simulink model "ModeloMotorMaxon"  (R2022b)
settings: Solver=VariableStepAuto  StartTime=0.0  StopTime=60  RelTol=1e-3
libraries: cstblocks x1, slident x1
settings Model: Creator=workstation  LastModifiedBy=workstation

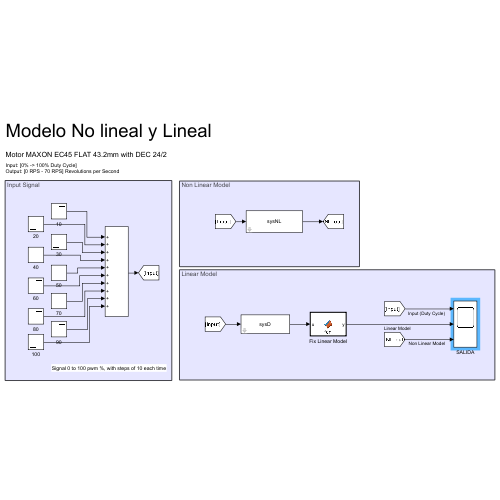
[thumbnail: Simulink's stored preview of the top-level diagram]
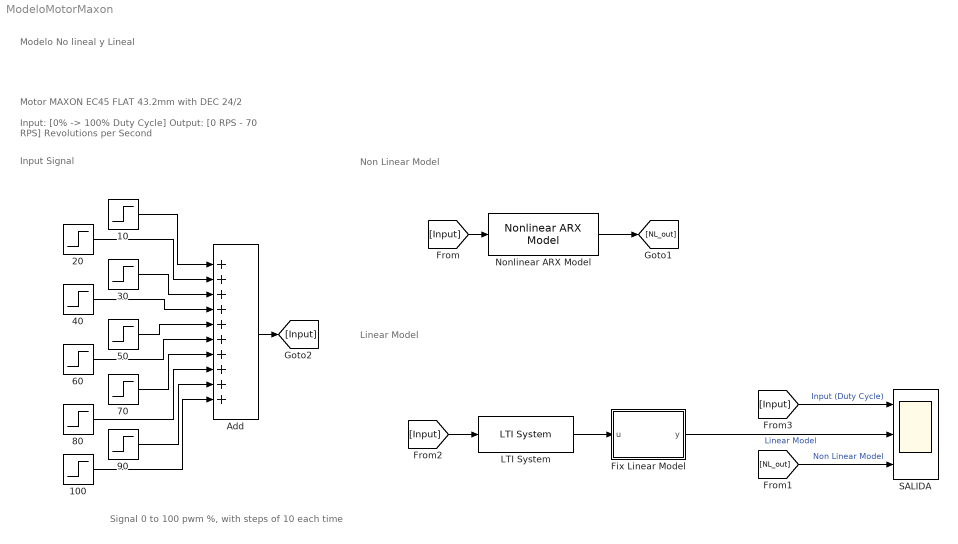
== system ModeloMotorMaxon ==
  note: Input: [0% -> 100% Duty Cycle]
      | Output: [0 RPS - 70 RPS] Revolutions per Second
  note: Signal 0 to 100 pwm %, with steps of 10 each time
  note: Input Signal
  note: Linear Model
  note: Non Linear Model
  note: Motor MAXON EC45 FLAT 43.2mm with DEC 24/2
  note: Modelo No lineal y Lineal
  10 : Step  Time=5  After=10  SampleTime=0
  100 : Step  Time=50  After=10  SampleTime=0
  20 : Step  Time=10  After=10  SampleTime=0
  30 : Step  Time=15  After=10  SampleTime=0
  40 : Step  Time=20  After=10  SampleTime=0
  50 : Step  Time=25  After=10  SampleTime=0
  60 : Step  Time=30  After=10  SampleTime=0
  70 : Step  Time=35  After=10  SampleTime=0
  80 : Step  Time=40  After=10  SampleTime=0
  90 : Step  Time=45  After=10  SampleTime=0
  Add : Sum  Inputs=++++++++++
  Fix Linear Model : MATLAB Function  TreatAsAtomicUnit=on
  LTI System : cstblocks/LTI System  sys=sysD  IC=[]
  Nonlinear ARX Model : slident/Models/Nonlinear ARX Model  sys=sysNL  ICspec=Input and output values  X0=0  U0=0  Y0=0
  SALIDA : Scope  NumInputPorts=3
  wires:
  Nonlinear ARX Model/1 -> [NL_out]
  LTI System/1 -> Fix Linear Model/1(u)
  Fix Linear Model/1(y) -> SALIDA/2  "Linear Model"
  [NL_out] -> SALIDA/3  "Non Linear Model"
  10/1 -> Add/1
  20/1 -> Add/2
  30/1 -> Add/3
  40/1 -> Add/4
  50/1 -> Add/5
  60/1 -> Add/6
  70/1 -> Add/7
  80/1 -> Add/8
  90/1 -> Add/9
  100/1 -> Add/10
  [Input] -> Nonlinear ARX Model/1
  [Input] -> LTI System/1
  Add/1 -> [Input]
  [Input] -> SALIDA/1  "Input (Duty Cycle)"

== matlab function ModeloMotorMaxon/Fix Linear Model ==
  data: u input; y output
function y = fcn(u)

yt=0;
if u > 5 % && u<10
    yt=u-7;
else
    yt=0;
end


y = yt;
